simulink model "ddc_bpm_476_066_bak6"  (Simulink 7.8)
settings: Solver=ode45  StartTime=0.0  StopTime=2.56e-3  RelTol=1e-3
undefined symbols (not defined in the file): dt_sim, frev_476, Fs_adc, xlipgetpartsetting
libraries: xbsIndex_r4 x615, simulink x3
(part 6 of 6)

== system ddc_bpm_476_066_bak6/delta-sigma_tbt/unsigned2signed1 ==
  s_data : Inport
  u_data : Inport  Port=2
  Concat : xbsIndex_r4/Concat  num_inputs=2  dbl_ovrd=off  block_type=concat
  Convert : xbsIndex_r4/Convert  gui_display_data_type=Fixed-point  arith_type="Signed  (2's comp)"  n_bits=24  bin_pt=23  float_type=Single  exp_bits=8  fraction_bits=24  quantization=Truncate  overflow=Flag as error  en=off  latency=0  dbl_ovrd=off  pipeline=off  block_type=convert
  Reinterpret : xbsIndex_r4/Reinterpret  force_arith_type=on  arith_type="Signed  (2's comp)"  force_bin_pt=on  bin_pt=23  block_type=reinterpret
  Reinterpret1 : xbsIndex_r4/Reinterpret  force_arith_type=on  arith_type=Unsigned  force_bin_pt=on  bin_pt=0  block_type=reinterpret
  Reinterpret2 : xbsIndex_r4/Reinterpret  force_arith_type=on  arith_type=Unsigned  force_bin_pt=on  bin_pt=0  block_type=reinterpret
  data_out : Outport
  wires:
  Concat/1 -> Reinterpret/1
  Reinterpret2/1 -> Concat/1
  s_data/1 -> Reinterpret2/1
  Reinterpret/1 -> Convert/1
  u_data/1 -> Reinterpret1/1
  Reinterpret1/1 -> Concat/2
  Convert/1 -> data_out/1

== system ddc_bpm_476_066_bak6/delta-sigma_tbt/unsigned2signed2 ==
  s_data : Inport
  u_data : Inport  Port=2
  Concat : xbsIndex_r4/Concat  num_inputs=2  dbl_ovrd=off  block_type=concat
  Convert : xbsIndex_r4/Convert  gui_display_data_type=Fixed-point  arith_type="Signed  (2's comp)"  n_bits=24  bin_pt=23  float_type=Single  exp_bits=8  fraction_bits=24  quantization=Truncate  overflow=Flag as error  en=off  latency=0  dbl_ovrd=off  pipeline=off  block_type=convert
  Reinterpret : xbsIndex_r4/Reinterpret  force_arith_type=on  arith_type="Signed  (2's comp)"  force_bin_pt=on  bin_pt=23  block_type=reinterpret
  Reinterpret1 : xbsIndex_r4/Reinterpret  force_arith_type=on  arith_type=Unsigned  force_bin_pt=on  bin_pt=0  block_type=reinterpret
  Reinterpret2 : xbsIndex_r4/Reinterpret  force_arith_type=on  arith_type=Unsigned  force_bin_pt=on  bin_pt=0  block_type=reinterpret
  data_out : Outport
  wires:
  Concat/1 -> Reinterpret/1
  Reinterpret2/1 -> Concat/1
  s_data/1 -> Reinterpret2/1
  Reinterpret/1 -> Convert/1
  u_data/1 -> Reinterpret1/1
  Reinterpret1/1 -> Concat/2
  Convert/1 -> data_out/1

== system ddc_bpm_476_066_bak6/delta-sigma_tbt/unsigned2signed3 ==
  s_data : Inport
  u_data : Inport  Port=2
  Concat : xbsIndex_r4/Concat  num_inputs=2  dbl_ovrd=off  block_type=concat
  Convert : xbsIndex_r4/Convert  gui_display_data_type=Fixed-point  arith_type="Signed  (2's comp)"  n_bits=24  bin_pt=23  float_type=Single  exp_bits=8  fraction_bits=24  quantization=Truncate  overflow=Flag as error  en=off  latency=0  dbl_ovrd=off  pipeline=off  block_type=convert
  Reinterpret : xbsIndex_r4/Reinterpret  force_arith_type=on  arith_type="Signed  (2's comp)"  force_bin_pt=on  bin_pt=23  block_type=reinterpret
  Reinterpret1 : xbsIndex_r4/Reinterpret  force_arith_type=on  arith_type=Unsigned  force_bin_pt=on  bin_pt=0  block_type=reinterpret
  Reinterpret2 : xbsIndex_r4/Reinterpret  force_arith_type=on  arith_type=Unsigned  force_bin_pt=on  bin_pt=0  block_type=reinterpret
  data_out : Outport
  wires:
  Concat/1 -> Reinterpret/1
  Reinterpret2/1 -> Concat/1
  s_data/1 -> Reinterpret2/1
  Reinterpret/1 -> Convert/1
  u_data/1 -> Reinterpret1/1
  Reinterpret1/1 -> Concat/2
  Convert/1 -> data_out/1

== system ddc_bpm_476_066_bak6/Channel0_tbt/DDC/Mixer ==
  din_q : Inport
  din_i : Inport  Port=2
  en : Inport  Port=3
  dds_valid : Inport  Port=4
  dds_cosine : Inport  Port=5
  dds_msine : Inport  Port=6
  ComplexMult : xbsIndex_r4/Complex Multiplier 5.0   hasatlast=off  hasatuser=off  atuserwidth=1  hasbtlast=off  hasbtuser=off  btuserwidth=1  multtype=Use_Mults  optimizegoal=Performance  flowcontrol=NonBlocking  outputwidth=24  roundmode=Truncate  hasctrltlast=off  hasctrltuser=off  ctrltuserwidth=1  outtlastbehv=Null  latencyconfig=Manual  minimumlatency=6  aclken=off  aresetn=off  trim_axipin_name=on  aportwidth=63  bportwidth=63  ip_name=Complex Multiplier  ip_version=5.0  dsptool_ready=true  ipcore_usecache=true  ipcore_useipmodelcache=true  ipcore_verbose=false  ipcore_latency_parameter='minimumlatency'  wrapper_available=true  port_translation_map={ 'aclken' => 'en', 'aresetn' => 'rst'}  structural_sim=false  block_type=cmpy_v5_0
  Convert1 : xbsIndex_r4/Convert  gui_display_data_type=Fixed-point  arith_type="Signed  (2's comp)"  n_bits=24  bin_pt=22  float_type=Single  exp_bits=8  fraction_bits=24  quantization=Truncate  overflow=Flag as error  en=off  latency=0  dbl_ovrd=off  pipeline=off  block_type=convert
  Convert2 : xbsIndex_r4/Convert  gui_display_data_type=Fixed-point  arith_type="Signed  (2's comp)"  n_bits=24  bin_pt=22  float_type=Single  exp_bits=8  fraction_bits=24  quantization=Truncate  overflow=Flag as error  en=off  latency=0  dbl_ovrd=off  pipeline=off  block_type=convert
  DataReg_En : Subsystem
  DataReg_En1 : Subsystem
  Delay : xbsIndex_r4/Delay  rst=off  infoeditControl=Selection of Reset will increase slice count due to use of real FFs and instead of SRLs  en=off  latency=0  dbl_ovrd=off  reg_retiming=off  block_type=delay
      settings: infoedit=Hardware notes: A delay line is a chain, each link of which is an SRL16 followed by a flip-flop. If register retiming is enabled, the delay line is a chain of flip-flops.  xl_area=[7 14 0 0 0 0 0]  block_version=VER_STRING_GOES_HERE
  Delay1 : xbsIndex_r4/Delay  rst=off  infoeditControl=Selection of Reset will increase slice count due to use of real FFs and instead of SRLs  en=off  latency=0  dbl_ovrd=off  reg_retiming=off  block_type=delay
      settings: infoedit=Hardware notes: A delay line is a chain, each link of which is an SRL16 followed by a flip-flop. If register retiming is enabled, the delay line is a chain of flip-flops.  xl_area=[7 14 0 0 0 0 0]  block_version=VER_STRING_GOES_HERE
  Delay{2..3,6..7} (4 alike) : xbsIndex_r4/Delay  rst=off  infoeditControl=Selection of Reset will increase slice count due to use of real FFs and instead of SRLs  en=on  latency=1  dbl_ovrd=off  reg_retiming=off  block_type=delay
  Reinterpret : xbsIndex_r4/Reinterpret  force_arith_type=off  arith_type=Unsigned  force_bin_pt=off  bin_pt=22  block_type=reinterpret
  Reinterpret1 : xbsIndex_r4/Reinterpret  force_arith_type=off  arith_type=Unsigned  force_bin_pt=off  bin_pt=22  block_type=reinterpret
  Q : Outport
  I : Outport  Port=2
  valid_out : Outport  Port=3
  wires:
  din_q/1 -> DataReg_En/1(Din)
  DataReg_En/1(Dout) -> Delay/1
  din_i/1 -> DataReg_En1/1(Din)
  DataReg_En1/1(Dout) -> Delay1/1
  en/1 -> DataReg_En/2(en), DataReg_En1/2(en)
  dds_cosine/1 -> Delay3/1
  dds_msine/1 -> Delay2/1
  Delay3/1 -> ComplexMult/3  "a_r"
  Delay6/1 -> Q/1
  Delay2/1 -> ComplexMult/2  "a_i"
  ComplexMult/2 -> Reinterpret/1
  ComplexMult/3 -> Reinterpret1/1
  ComplexMult/1 -> Delay7/2, Delay6/2
  Delay1/1 -> ComplexMult/6  "b_r"
  Delay/1 -> ComplexMult/5  "b_i"
  DataReg_En/2(Valid) -> ComplexMult/4
  Delay7/1 -> I/1
  DataReg_En1/2(Valid) -> valid_out/1
  Convert1/1 -> Delay7/1
  Convert2/1 -> Delay6/1
  Reinterpret/1 -> Convert2/1
  Reinterpret1/1 -> Convert1/1
  dds_valid/1 -> Delay2/2, Delay3/2, ComplexMult/1

== system ddc_bpm_476_066_bak6/Channel0_tbt/decim35/Cast1 ==
  data_in : Inport
  en : Inport  Port=2
  Register : xbsIndex_r4/Register  init=0  rst=off  en=on  dbl_ovrd=off  block_type=register
      settings: xl_area=[0, 0, 0, 0, 0, 0, 0]  block_version=VER_STRING_GOES_HERE
  Register1 : xbsIndex_r4/Register  init=0  rst=off  en=off  dbl_ovrd=off  block_type=register
      settings: xl_area=[0, 0, 0, 0, 0, 0, 0]  block_version=VER_STRING_GOES_HERE
  format1 : Subsystem
  out : Outport
  valid : Outport  Port=2
  wires:
  format1/1(dout) -> Register/1
  Register/1 -> out/1
  data_in/1 -> format1/1(din)
  en/1 -> Register/2, Register1/1
  Register1/1 -> valid/1

== system ddc_bpm_476_066_bak6/Channel0_tbt/decim35/Cast4 ==
  data_in : Inport
  en : Inport  Port=2
  Register : xbsIndex_r4/Register  init=0  rst=off  en=on  dbl_ovrd=off  block_type=register
      settings: xl_area=[0, 0, 0, 0, 0, 0, 0]  block_version=VER_STRING_GOES_HERE
  Register1 : xbsIndex_r4/Register  init=0  rst=off  en=off  dbl_ovrd=off  block_type=register
      settings: xl_area=[0, 0, 0, 0, 0, 0, 0]  block_version=VER_STRING_GOES_HERE
  format1 : Subsystem
  out : Outport
  valid : Outport  Port=2
  wires:
  format1/1(dout) -> Register/1
  Register/1 -> out/1
  data_in/1 -> format1/1(din)
  en/1 -> Register/2, Register1/1
  Register1/1 -> valid/1

== system ddc_bpm_476_066_bak6/Channel1_tbt/DDC/Mixer ==
  din_q : Inport
  din_i : Inport  Port=2
  en : Inport  Port=3
  dds_valid : Inport  Port=4
  dds_cosine : Inport  Port=5
  dds_msine : Inport  Port=6
  ComplexMult : xbsIndex_r4/Complex Multiplier 5.0   hasatlast=off  hasatuser=off  atuserwidth=1  hasbtlast=off  hasbtuser=off  btuserwidth=1  multtype=Use_Mults  optimizegoal=Performance  flowcontrol=NonBlocking  outputwidth=24  roundmode=Truncate  hasctrltlast=off  hasctrltuser=off  ctrltuserwidth=1  outtlastbehv=Null  latencyconfig=Manual  minimumlatency=6  aclken=off  aresetn=off  trim_axipin_name=on  aportwidth=63  bportwidth=63  ip_name=Complex Multiplier  ip_version=5.0  dsptool_ready=true  ipcore_usecache=true  ipcore_useipmodelcache=true  ipcore_verbose=false  ipcore_latency_parameter='minimumlatency'  wrapper_available=true  port_translation_map={ 'aclken' => 'en', 'aresetn' => 'rst'}  structural_sim=false  block_type=cmpy_v5_0
  Convert1 : xbsIndex_r4/Convert  gui_display_data_type=Fixed-point  arith_type="Signed  (2's comp)"  n_bits=24  bin_pt=22  float_type=Single  exp_bits=8  fraction_bits=24  quantization=Truncate  overflow=Flag as error  en=off  latency=0  dbl_ovrd=off  pipeline=off  block_type=convert
  Convert2 : xbsIndex_r4/Convert  gui_display_data_type=Fixed-point  arith_type="Signed  (2's comp)"  n_bits=24  bin_pt=22  float_type=Single  exp_bits=8  fraction_bits=24  quantization=Truncate  overflow=Flag as error  en=off  latency=0  dbl_ovrd=off  pipeline=off  block_type=convert
  DataReg_En : Subsystem
  DataReg_En1 : Subsystem
  Delay : xbsIndex_r4/Delay  rst=off  infoeditControl=Selection of Reset will increase slice count due to use of real FFs and instead of SRLs  en=off  latency=0  dbl_ovrd=off  reg_retiming=off  block_type=delay
      settings: infoedit=Hardware notes: A delay line is a chain, each link of which is an SRL16 followed by a flip-flop. If register retiming is enabled, the delay line is a chain of flip-flops.  xl_area=[7 14 0 0 0 0 0]  block_version=VER_STRING_GOES_HERE
  Delay1 : xbsIndex_r4/Delay  rst=off  infoeditControl=Selection of Reset will increase slice count due to use of real FFs and instead of SRLs  en=off  latency=0  dbl_ovrd=off  reg_retiming=off  block_type=delay
      settings: infoedit=Hardware notes: A delay line is a chain, each link of which is an SRL16 followed by a flip-flop. If register retiming is enabled, the delay line is a chain of flip-flops.  xl_area=[7 14 0 0 0 0 0]  block_version=VER_STRING_GOES_HERE
  Delay{2..3,6..7} (4 alike) : xbsIndex_r4/Delay  rst=off  infoeditControl=Selection of Reset will increase slice count due to use of real FFs and instead of SRLs  en=on  latency=1  dbl_ovrd=off  reg_retiming=off  block_type=delay
  Reinterpret : xbsIndex_r4/Reinterpret  force_arith_type=off  arith_type=Unsigned  force_bin_pt=off  bin_pt=22  block_type=reinterpret
  Reinterpret1 : xbsIndex_r4/Reinterpret  force_arith_type=off  arith_type=Unsigned  force_bin_pt=off  bin_pt=22  block_type=reinterpret
  Q : Outport
  I : Outport  Port=2
  valid_out : Outport  Port=3
  wires:
  din_q/1 -> DataReg_En/1(Din)
  DataReg_En/1(Dout) -> Delay/1
  din_i/1 -> DataReg_En1/1(Din)
  DataReg_En1/1(Dout) -> Delay1/1
  en/1 -> DataReg_En/2(en), DataReg_En1/2(en)
  dds_cosine/1 -> Delay3/1
  dds_msine/1 -> Delay2/1
  Delay3/1 -> ComplexMult/3  "a_r"
  Delay6/1 -> Q/1
  Delay2/1 -> ComplexMult/2  "a_i"
  ComplexMult/2 -> Reinterpret/1
  ComplexMult/3 -> Reinterpret1/1
  ComplexMult/1 -> Delay7/2, Delay6/2
  Delay1/1 -> ComplexMult/6  "b_r"
  Delay/1 -> ComplexMult/5  "b_i"
  DataReg_En/2(Valid) -> ComplexMult/4
  Delay7/1 -> I/1
  DataReg_En1/2(Valid) -> valid_out/1
  Convert1/1 -> Delay7/1
  Convert2/1 -> Delay6/1
  Reinterpret/1 -> Convert2/1
  Reinterpret1/1 -> Convert1/1
  dds_valid/1 -> Delay2/2, Delay3/2, ComplexMult/1

== system ddc_bpm_476_066_bak6/Channel1_tbt/decim35/Cast1 ==
  data_in : Inport
  en : Inport  Port=2
  Register : xbsIndex_r4/Register  init=0  rst=off  en=on  dbl_ovrd=off  block_type=register
      settings: xl_area=[0, 0, 0, 0, 0, 0, 0]  block_version=VER_STRING_GOES_HERE
  Register1 : xbsIndex_r4/Register  init=0  rst=off  en=off  dbl_ovrd=off  block_type=register
      settings: xl_area=[0, 0, 0, 0, 0, 0, 0]  block_version=VER_STRING_GOES_HERE
  format1 : Subsystem
  out : Outport
  valid : Outport  Port=2
  wires:
  format1/1(dout) -> Register/1
  Register/1 -> out/1
  data_in/1 -> format1/1(din)
  en/1 -> Register/2, Register1/1
  Register1/1 -> valid/1

== system ddc_bpm_476_066_bak6/Channel1_tbt/decim35/Cast4 ==
  data_in : Inport
  en : Inport  Port=2
  Register : xbsIndex_r4/Register  init=0  rst=off  en=on  dbl_ovrd=off  block_type=register
      settings: xl_area=[0, 0, 0, 0, 0, 0, 0]  block_version=VER_STRING_GOES_HERE
  Register1 : xbsIndex_r4/Register  init=0  rst=off  en=off  dbl_ovrd=off  block_type=register
      settings: xl_area=[0, 0, 0, 0, 0, 0, 0]  block_version=VER_STRING_GOES_HERE
  format1 : Subsystem
  out : Outport
  valid : Outport  Port=2
  wires:
  format1/1(dout) -> Register/1
  Register/1 -> out/1
  data_in/1 -> format1/1(din)
  en/1 -> Register/2, Register1/1
  Register1/1 -> valid/1

== system ddc_bpm_476_066_bak6/Channel2_tbt/DDC/Mixer ==
  din_q : Inport
  din_i : Inport  Port=2
  en : Inport  Port=3
  dds_valid : Inport  Port=4
  dds_cosine : Inport  Port=5
  dds_msine : Inport  Port=6
  ComplexMult : xbsIndex_r4/Complex Multiplier 5.0   hasatlast=off  hasatuser=off  atuserwidth=1  hasbtlast=off  hasbtuser=off  btuserwidth=1  multtype=Use_Mults  optimizegoal=Performance  flowcontrol=NonBlocking  outputwidth=24  roundmode=Truncate  hasctrltlast=off  hasctrltuser=off  ctrltuserwidth=1  outtlastbehv=Null  latencyconfig=Manual  minimumlatency=6  aclken=off  aresetn=off  trim_axipin_name=on  aportwidth=63  bportwidth=63  ip_name=Complex Multiplier  ip_version=5.0  dsptool_ready=true  ipcore_usecache=true  ipcore_useipmodelcache=true  ipcore_verbose=false  ipcore_latency_parameter='minimumlatency'  wrapper_available=true  port_translation_map={ 'aclken' => 'en', 'aresetn' => 'rst'}  structural_sim=false  block_type=cmpy_v5_0
  Convert1 : xbsIndex_r4/Convert  gui_display_data_type=Fixed-point  arith_type="Signed  (2's comp)"  n_bits=24  bin_pt=22  float_type=Single  exp_bits=8  fraction_bits=24  quantization=Truncate  overflow=Flag as error  en=off  latency=0  dbl_ovrd=off  pipeline=off  block_type=convert
  Convert2 : xbsIndex_r4/Convert  gui_display_data_type=Fixed-point  arith_type="Signed  (2's comp)"  n_bits=24  bin_pt=22  float_type=Single  exp_bits=8  fraction_bits=24  quantization=Truncate  overflow=Flag as error  en=off  latency=0  dbl_ovrd=off  pipeline=off  block_type=convert
  DataReg_En : Subsystem
  DataReg_En1 : Subsystem
  Delay : xbsIndex_r4/Delay  rst=off  infoeditControl=Selection of Reset will increase slice count due to use of real FFs and instead of SRLs  en=off  latency=0  dbl_ovrd=off  reg_retiming=off  block_type=delay
      settings: infoedit=Hardware notes: A delay line is a chain, each link of which is an SRL16 followed by a flip-flop. If register retiming is enabled, the delay line is a chain of flip-flops.  xl_area=[7 14 0 0 0 0 0]  block_version=VER_STRING_GOES_HERE
  Delay1 : xbsIndex_r4/Delay  rst=off  infoeditControl=Selection of Reset will increase slice count due to use of real FFs and instead of SRLs  en=off  latency=0  dbl_ovrd=off  reg_retiming=off  block_type=delay
      settings: infoedit=Hardware notes: A delay line is a chain, each link of which is an SRL16 followed by a flip-flop. If register retiming is enabled, the delay line is a chain of flip-flops.  xl_area=[7 14 0 0 0 0 0]  block_version=VER_STRING_GOES_HERE
  Delay{2..3,6..7} (4 alike) : xbsIndex_r4/Delay  rst=off  infoeditControl=Selection of Reset will increase slice count due to use of real FFs and instead of SRLs  en=on  latency=1  dbl_ovrd=off  reg_retiming=off  block_type=delay
  Reinterpret : xbsIndex_r4/Reinterpret  force_arith_type=off  arith_type=Unsigned  force_bin_pt=off  bin_pt=22  block_type=reinterpret
  Reinterpret1 : xbsIndex_r4/Reinterpret  force_arith_type=off  arith_type=Unsigned  force_bin_pt=off  bin_pt=22  block_type=reinterpret
  Q : Outport
  I : Outport  Port=2
  valid_out : Outport  Port=3
  wires:
  din_q/1 -> DataReg_En/1(Din)
  DataReg_En/1(Dout) -> Delay/1
  din_i/1 -> DataReg_En1/1(Din)
  DataReg_En1/1(Dout) -> Delay1/1
  en/1 -> DataReg_En/2(en), DataReg_En1/2(en)
  dds_cosine/1 -> Delay3/1
  dds_msine/1 -> Delay2/1
  Delay3/1 -> ComplexMult/3  "a_r"
  Delay6/1 -> Q/1
  Delay2/1 -> ComplexMult/2  "a_i"
  ComplexMult/2 -> Reinterpret/1
  ComplexMult/3 -> Reinterpret1/1
  ComplexMult/1 -> Delay7/2, Delay6/2
  Delay1/1 -> ComplexMult/6  "b_r"
  Delay/1 -> ComplexMult/5  "b_i"
  DataReg_En/2(Valid) -> ComplexMult/4
  Delay7/1 -> I/1
  DataReg_En1/2(Valid) -> valid_out/1
  Convert1/1 -> Delay7/1
  Convert2/1 -> Delay6/1
  Reinterpret/1 -> Convert2/1
  Reinterpret1/1 -> Convert1/1
  dds_valid/1 -> Delay2/2, Delay3/2, ComplexMult/1

== system ddc_bpm_476_066_bak6/Channel2_tbt/decim35/Cast1 ==
  data_in : Inport
  en : Inport  Port=2
  Register : xbsIndex_r4/Register  init=0  rst=off  en=on  dbl_ovrd=off  block_type=register
      settings: xl_area=[0, 0, 0, 0, 0, 0, 0]  block_version=VER_STRING_GOES_HERE
  Register1 : xbsIndex_r4/Register  init=0  rst=off  en=off  dbl_ovrd=off  block_type=register
      settings: xl_area=[0, 0, 0, 0, 0, 0, 0]  block_version=VER_STRING_GOES_HERE
  format1 : Subsystem
  out : Outport
  valid : Outport  Port=2
  wires:
  format1/1(dout) -> Register/1
  Register/1 -> out/1
  data_in/1 -> format1/1(din)
  en/1 -> Register/2, Register1/1
  Register1/1 -> valid/1

== system ddc_bpm_476_066_bak6/Channel2_tbt/decim35/Cast4 ==
  data_in : Inport
  en : Inport  Port=2
  Register : xbsIndex_r4/Register  init=0  rst=off  en=on  dbl_ovrd=off  block_type=register
      settings: xl_area=[0, 0, 0, 0, 0, 0, 0]  block_version=VER_STRING_GOES_HERE
  Register1 : xbsIndex_r4/Register  init=0  rst=off  en=off  dbl_ovrd=off  block_type=register
      settings: xl_area=[0, 0, 0, 0, 0, 0, 0]  block_version=VER_STRING_GOES_HERE
  format1 : Subsystem
  out : Outport
  valid : Outport  Port=2
  wires:
  format1/1(dout) -> Register/1
  Register/1 -> out/1
  data_in/1 -> format1/1(din)
  en/1 -> Register/2, Register1/1
  Register1/1 -> valid/1

== system ddc_bpm_476_066_bak6/Channel3_tbt/DDC/Mixer ==
  din_q : Inport
  din_i : Inport  Port=2
  en : Inport  Port=3
  dds_valid : Inport  Port=4
  dds_cosine : Inport  Port=5
  dds_msine : Inport  Port=6
  ComplexMult : xbsIndex_r4/Complex Multiplier 5.0   hasatlast=off  hasatuser=off  atuserwidth=1  hasbtlast=off  hasbtuser=off  btuserwidth=1  multtype=Use_Mults  optimizegoal=Performance  flowcontrol=NonBlocking  outputwidth=24  roundmode=Truncate  hasctrltlast=off  hasctrltuser=off  ctrltuserwidth=1  outtlastbehv=Null  latencyconfig=Manual  minimumlatency=6  aclken=off  aresetn=off  trim_axipin_name=on  aportwidth=63  bportwidth=63  ip_name=Complex Multiplier  ip_version=5.0  dsptool_ready=true  ipcore_usecache=true  ipcore_useipmodelcache=true  ipcore_verbose=false  ipcore_latency_parameter='minimumlatency'  wrapper_available=true  port_translation_map={ 'aclken' => 'en', 'aresetn' => 'rst'}  structural_sim=false  block_type=cmpy_v5_0
  Convert1 : xbsIndex_r4/Convert  gui_display_data_type=Fixed-point  arith_type="Signed  (2's comp)"  n_bits=24  bin_pt=22  float_type=Single  exp_bits=8  fraction_bits=24  quantization=Truncate  overflow=Flag as error  en=off  latency=0  dbl_ovrd=off  pipeline=off  block_type=convert
  Convert2 : xbsIndex_r4/Convert  gui_display_data_type=Fixed-point  arith_type="Signed  (2's comp)"  n_bits=24  bin_pt=22  float_type=Single  exp_bits=8  fraction_bits=24  quantization=Truncate  overflow=Flag as error  en=off  latency=0  dbl_ovrd=off  pipeline=off  block_type=convert
  DataReg_En : Subsystem
  DataReg_En1 : Subsystem
  Delay : xbsIndex_r4/Delay  rst=off  infoeditControl=Selection of Reset will increase slice count due to use of real FFs and instead of SRLs  en=off  latency=0  dbl_ovrd=off  reg_retiming=off  block_type=delay
      settings: infoedit=Hardware notes: A delay line is a chain, each link of which is an SRL16 followed by a flip-flop. If register retiming is enabled, the delay line is a chain of flip-flops.  xl_area=[7 14 0 0 0 0 0]  block_version=VER_STRING_GOES_HERE
  Delay1 : xbsIndex_r4/Delay  rst=off  infoeditControl=Selection of Reset will increase slice count due to use of real FFs and instead of SRLs  en=off  latency=0  dbl_ovrd=off  reg_retiming=off  block_type=delay
      settings: infoedit=Hardware notes: A delay line is a chain, each link of which is an SRL16 followed by a flip-flop. If register retiming is enabled, the delay line is a chain of flip-flops.  xl_area=[7 14 0 0 0 0 0]  block_version=VER_STRING_GOES_HERE
  Delay{2..3,6..7} (4 alike) : xbsIndex_r4/Delay  rst=off  infoeditControl=Selection of Reset will increase slice count due to use of real FFs and instead of SRLs  en=on  latency=1  dbl_ovrd=off  reg_retiming=off  block_type=delay
  Reinterpret : xbsIndex_r4/Reinterpret  force_arith_type=off  arith_type=Unsigned  force_bin_pt=off  bin_pt=22  block_type=reinterpret
  Reinterpret1 : xbsIndex_r4/Reinterpret  force_arith_type=off  arith_type=Unsigned  force_bin_pt=off  bin_pt=22  block_type=reinterpret
  Q : Outport
  I : Outport  Port=2
  valid_out : Outport  Port=3
  wires:
  din_q/1 -> DataReg_En/1(Din)
  DataReg_En/1(Dout) -> Delay/1
  din_i/1 -> DataReg_En1/1(Din)
  DataReg_En1/1(Dout) -> Delay1/1
  en/1 -> DataReg_En/2(en), DataReg_En1/2(en)
  dds_cosine/1 -> Delay3/1
  dds_msine/1 -> Delay2/1
  Delay3/1 -> ComplexMult/3  "a_r"
  Delay6/1 -> Q/1
  Delay2/1 -> ComplexMult/2  "a_i"
  ComplexMult/2 -> Reinterpret/1
  ComplexMult/3 -> Reinterpret1/1
  ComplexMult/1 -> Delay7/2, Delay6/2
  Delay1/1 -> ComplexMult/6  "b_r"
  Delay/1 -> ComplexMult/5  "b_i"
  DataReg_En/2(Valid) -> ComplexMult/4
  Delay7/1 -> I/1
  DataReg_En1/2(Valid) -> valid_out/1
  Convert1/1 -> Delay7/1
  Convert2/1 -> Delay6/1
  Reinterpret/1 -> Convert2/1
  Reinterpret1/1 -> Convert1/1
  dds_valid/1 -> Delay2/2, Delay3/2, ComplexMult/1

== system ddc_bpm_476_066_bak6/Channel3_tbt/decim35/Cast1 ==
  data_in : Inport
  en : Inport  Port=2
  Register : xbsIndex_r4/Register  init=0  rst=off  en=on  dbl_ovrd=off  block_type=register
      settings: xl_area=[0, 0, 0, 0, 0, 0, 0]  block_version=VER_STRING_GOES_HERE
  Register1 : xbsIndex_r4/Register  init=0  rst=off  en=off  dbl_ovrd=off  block_type=register
      settings: xl_area=[0, 0, 0, 0, 0, 0, 0]  block_version=VER_STRING_GOES_HERE
  format1 : Subsystem
  out : Outport
  valid : Outport  Port=2
  wires:
  format1/1(dout) -> Register/1
  Register/1 -> out/1
  data_in/1 -> format1/1(din)
  en/1 -> Register/2, Register1/1
  Register1/1 -> valid/1

== system ddc_bpm_476_066_bak6/Channel3_tbt/decim35/Cast4 ==
  data_in : Inport
  en : Inport  Port=2
  Register : xbsIndex_r4/Register  init=0  rst=off  en=on  dbl_ovrd=off  block_type=register
      settings: xl_area=[0, 0, 0, 0, 0, 0, 0]  block_version=VER_STRING_GOES_HERE
  Register1 : xbsIndex_r4/Register  init=0  rst=off  en=off  dbl_ovrd=off  block_type=register
      settings: xl_area=[0, 0, 0, 0, 0, 0, 0]  block_version=VER_STRING_GOES_HERE
  format1 : Subsystem
  out : Outport
  valid : Outport  Port=2
  wires:
  format1/1(dout) -> Register/1
  Register/1 -> out/1
  data_in/1 -> format1/1(din)
  en/1 -> Register/2, Register1/1
  Register1/1 -> valid/1

== system ddc_bpm_476_066_bak6/Decim_monit/Cast/format1 ==
  din : Inport
  Convert : xbsIndex_r4/Convert  gui_display_data_type=Fixed-point  arith_type="Signed  (2's comp)"  n_bits=24  bin_pt=22  float_type=Single  exp_bits=8  fraction_bits=24  quantization="Round  (unbiased: +/- Inf)"  overflow=Flag as error  en=off  latency=0  dbl_ovrd=off  pipeline=off  block_type=convert
  Reinterpret : xbsIndex_r4/Reinterpret  force_arith_type=on  arith_type="Signed  (2's comp)"  force_bin_pt=off  bin_pt=22  block_type=reinterpret
      settings: block_version=10.1
  dout : Outport
  wires:
  din/1 -> Reinterpret/1
  Convert/1 -> dout/1
  Reinterpret/1 -> Convert/1

== system ddc_bpm_476_066_bak6/Decim_monit/Cast1/format1 ==
  din : Inport
  Convert : xbsIndex_r4/Convert  gui_display_data_type=Fixed-point  arith_type="Signed  (2's comp)"  n_bits=24  bin_pt=22  float_type=Single  exp_bits=8  fraction_bits=24  quantization="Round  (unbiased: +/- Inf)"  overflow=Flag as error  en=off  latency=0  dbl_ovrd=off  pipeline=off  block_type=convert
  Reinterpret : xbsIndex_r4/Reinterpret  force_arith_type=on  arith_type="Signed  (2's comp)"  force_bin_pt=off  bin_pt=22  block_type=reinterpret
      settings: block_version=10.1
  dout : Outport
  wires:
  din/1 -> Reinterpret/1
  Convert/1 -> dout/1
  Reinterpret/1 -> Convert/1

== system ddc_bpm_476_066_bak6/Decim_monit/Cast2/format1 ==
  din : Inport
  Convert : xbsIndex_r4/Convert  gui_display_data_type=Fixed-point  arith_type="Signed  (2's comp)"  n_bits=24  bin_pt=22  float_type=Single  exp_bits=8  fraction_bits=24  quantization="Round  (unbiased: +/- Inf)"  overflow=Flag as error  en=off  latency=0  dbl_ovrd=off  pipeline=off  block_type=convert
  Reinterpret : xbsIndex_r4/Reinterpret  force_arith_type=on  arith_type="Signed  (2's comp)"  force_bin_pt=off  bin_pt=22  block_type=reinterpret
      settings: block_version=10.1
  dout : Outport
  wires:
  din/1 -> Reinterpret/1
  Convert/1 -> dout/1
  Reinterpret/1 -> Convert/1

== system ddc_bpm_476_066_bak6/Decim_monit/Cast3/format1 ==
  din : Inport
  Convert : xbsIndex_r4/Convert  gui_display_data_type=Fixed-point  arith_type="Signed  (2's comp)"  n_bits=24  bin_pt=22  float_type=Single  exp_bits=8  fraction_bits=24  quantization="Round  (unbiased: +/- Inf)"  overflow=Flag as error  en=off  latency=0  dbl_ovrd=off  pipeline=off  block_type=convert
  Reinterpret : xbsIndex_r4/Reinterpret  force_arith_type=on  arith_type="Signed  (2's comp)"  force_bin_pt=off  bin_pt=22  block_type=reinterpret
      settings: block_version=10.1
  dout : Outport
  wires:
  din/1 -> Reinterpret/1
  Convert/1 -> dout/1
  Reinterpret/1 -> Convert/1

== system ddc_bpm_476_066_bak6/Decim_monit/Cast4/format1 ==
  din : Inport
  Convert : xbsIndex_r4/Convert  gui_display_data_type=Fixed-point  arith_type="Signed  (2's comp)"  n_bits=24  bin_pt=22  float_type=Single  exp_bits=8  fraction_bits=24  quantization="Round  (unbiased: +/- Inf)"  overflow=Flag as error  en=off  latency=0  dbl_ovrd=off  pipeline=off  block_type=convert
  Reinterpret : xbsIndex_r4/Reinterpret  force_arith_type=on  arith_type="Signed  (2's comp)"  force_bin_pt=off  bin_pt=22  block_type=reinterpret
      settings: block_version=10.1
  dout : Outport
  wires:
  din/1 -> Reinterpret/1
  Convert/1 -> dout/1
  Reinterpret/1 -> Convert/1

== system ddc_bpm_476_066_bak6/Decim_monit/Cast5/format1 ==
  din : Inport
  Convert : xbsIndex_r4/Convert  gui_display_data_type=Fixed-point  arith_type="Signed  (2's comp)"  n_bits=24  bin_pt=22  float_type=Single  exp_bits=8  fraction_bits=24  quantization="Round  (unbiased: +/- Inf)"  overflow=Flag as error  en=off  latency=0  dbl_ovrd=off  pipeline=off  block_type=convert
  Reinterpret : xbsIndex_r4/Reinterpret  force_arith_type=on  arith_type="Signed  (2's comp)"  force_bin_pt=off  bin_pt=22  block_type=reinterpret
      settings: block_version=10.1
  dout : Outport
  wires:
  din/1 -> Reinterpret/1
  Convert/1 -> dout/1
  Reinterpret/1 -> Convert/1

== system ddc_bpm_476_066_bak6/Decim_monit/Cast6/format1 ==
  din : Inport
  Convert : xbsIndex_r4/Convert  gui_display_data_type=Fixed-point  arith_type="Signed  (2's comp)"  n_bits=24  bin_pt=22  float_type=Single  exp_bits=8  fraction_bits=24  quantization="Round  (unbiased: +/- Inf)"  overflow=Flag as error  en=off  latency=0  dbl_ovrd=off  pipeline=off  block_type=convert
  Reinterpret : xbsIndex_r4/Reinterpret  force_arith_type=on  arith_type="Signed  (2's comp)"  force_bin_pt=off  bin_pt=22  block_type=reinterpret
      settings: block_version=10.1
  dout : Outport
  wires:
  din/1 -> Reinterpret/1
  Convert/1 -> dout/1
  Reinterpret/1 -> Convert/1

== system ddc_bpm_476_066_bak6/Decim_monit/Cast7/format1 ==
  din : Inport
  Convert : xbsIndex_r4/Convert  gui_display_data_type=Fixed-point  arith_type="Signed  (2's comp)"  n_bits=24  bin_pt=22  float_type=Single  exp_bits=8  fraction_bits=24  quantization="Round  (unbiased: +/- Inf)"  overflow=Flag as error  en=off  latency=0  dbl_ovrd=off  pipeline=off  block_type=convert
  Reinterpret : xbsIndex_r4/Reinterpret  force_arith_type=on  arith_type="Signed  (2's comp)"  force_bin_pt=off  bin_pt=22  block_type=reinterpret
      settings: block_version=10.1
  dout : Outport
  wires:
  din/1 -> Reinterpret/1
  Convert/1 -> dout/1
  Reinterpret/1 -> Convert/1

== system ddc_bpm_476_066_bak6/Channel0_tbt/DDC/Mixer/DataReg_En ==
  Din : Inport
  en : Inport  Port=2
  Register : xbsIndex_r4/Register  init=0  rst=off  en=on  dbl_ovrd=off  block_type=register
      settings: block_version=VER_STRING_GOES_HERE
  Register1 : xbsIndex_r4/Register  init=0  rst=off  en=off  dbl_ovrd=off  block_type=register
      settings: block_version=VER_STRING_GOES_HERE
  Dout : Outport
  Valid : Outport  Port=2
  wires:
  Din/1 -> Register/1
  Register/1 -> Dout/1
  Register1/1 -> Valid/1
  en/1 -> Register1/1, Register/2

== system ddc_bpm_476_066_bak6/Channel0_tbt/DDC/Mixer/DataReg_En1 ==
  Din : Inport
  en : Inport  Port=2
  Register : xbsIndex_r4/Register  init=0  rst=off  en=on  dbl_ovrd=off  block_type=register
      settings: block_version=VER_STRING_GOES_HERE
  Register1 : xbsIndex_r4/Register  init=0  rst=off  en=off  dbl_ovrd=off  block_type=register
      settings: block_version=VER_STRING_GOES_HERE
  Dout : Outport
  Valid : Outport  Port=2
  wires:
  en/1 -> Register1/1, Register/2
  Register1/1 -> Valid/1
  Register/1 -> Dout/1
  Din/1 -> Register/1

== system ddc_bpm_476_066_bak6/Channel0_tbt/decim35/Cast1/format1 ==
  din : Inport
  Convert : xbsIndex_r4/Convert  gui_display_data_type=Fixed-point  arith_type="Signed  (2's comp)"  n_bits=24  bin_pt=22  float_type=Single  exp_bits=8  fraction_bits=24  quantization="Round  (unbiased: +/- Inf)"  overflow=Flag as error  en=off  latency=0  dbl_ovrd=off  pipeline=off  block_type=convert
  Reinterpret : xbsIndex_r4/Reinterpret  force_arith_type=on  arith_type="Signed  (2's comp)"  force_bin_pt=off  bin_pt=22  block_type=reinterpret
      settings: block_version=10.1
  dout : Outport
  wires:
  din/1 -> Reinterpret/1
  Convert/1 -> dout/1
  Reinterpret/1 -> Convert/1

== system ddc_bpm_476_066_bak6/Channel0_tbt/decim35/Cast4/format1 ==
  din : Inport
  Convert : xbsIndex_r4/Convert  gui_display_data_type=Fixed-point  arith_type="Signed  (2's comp)"  n_bits=24  bin_pt=22  float_type=Single  exp_bits=8  fraction_bits=24  quantization="Round  (unbiased: +/- Inf)"  overflow=Flag as error  en=off  latency=0  dbl_ovrd=off  pipeline=off  block_type=convert
  Reinterpret : xbsIndex_r4/Reinterpret  force_arith_type=on  arith_type="Signed  (2's comp)"  force_bin_pt=off  bin_pt=22  block_type=reinterpret
      settings: block_version=10.1
  dout : Outport
  wires:
  din/1 -> Reinterpret/1
  Convert/1 -> dout/1
  Reinterpret/1 -> Convert/1

== system ddc_bpm_476_066_bak6/Channel1_tbt/DDC/Mixer/DataReg_En ==
  Din : Inport
  en : Inport  Port=2
  Register : xbsIndex_r4/Register  init=0  rst=off  en=on  dbl_ovrd=off  block_type=register
      settings: block_version=VER_STRING_GOES_HERE
  Register1 : xbsIndex_r4/Register  init=0  rst=off  en=off  dbl_ovrd=off  block_type=register
      settings: block_version=VER_STRING_GOES_HERE
  Dout : Outport
  Valid : Outport  Port=2
  wires:
  Din/1 -> Register/1
  Register/1 -> Dout/1
  Register1/1 -> Valid/1
  en/1 -> Register1/1, Register/2

== system ddc_bpm_476_066_bak6/Channel1_tbt/DDC/Mixer/DataReg_En1 ==
  Din : Inport
  en : Inport  Port=2
  Register : xbsIndex_r4/Register  init=0  rst=off  en=on  dbl_ovrd=off  block_type=register
      settings: block_version=VER_STRING_GOES_HERE
  Register1 : xbsIndex_r4/Register  init=0  rst=off  en=off  dbl_ovrd=off  block_type=register
      settings: block_version=VER_STRING_GOES_HERE
  Dout : Outport
  Valid : Outport  Port=2
  wires:
  en/1 -> Register1/1, Register/2
  Register1/1 -> Valid/1
  Register/1 -> Dout/1
  Din/1 -> Register/1

== system ddc_bpm_476_066_bak6/Channel1_tbt/decim35/Cast1/format1 ==
  din : Inport
  Convert : xbsIndex_r4/Convert  gui_display_data_type=Fixed-point  arith_type="Signed  (2's comp)"  n_bits=24  bin_pt=22  float_type=Single  exp_bits=8  fraction_bits=24  quantization="Round  (unbiased: +/- Inf)"  overflow=Flag as error  en=off  latency=0  dbl_ovrd=off  pipeline=off  block_type=convert
  Reinterpret : xbsIndex_r4/Reinterpret  force_arith_type=on  arith_type="Signed  (2's comp)"  force_bin_pt=off  bin_pt=22  block_type=reinterpret
      settings: block_version=10.1
  dout : Outport
  wires:
  din/1 -> Reinterpret/1
  Convert/1 -> dout/1
  Reinterpret/1 -> Convert/1

== system ddc_bpm_476_066_bak6/Channel1_tbt/decim35/Cast4/format1 ==
  din : Inport
  Convert : xbsIndex_r4/Convert  gui_display_data_type=Fixed-point  arith_type="Signed  (2's comp)"  n_bits=24  bin_pt=22  float_type=Single  exp_bits=8  fraction_bits=24  quantization="Round  (unbiased: +/- Inf)"  overflow=Flag as error  en=off  latency=0  dbl_ovrd=off  pipeline=off  block_type=convert
  Reinterpret : xbsIndex_r4/Reinterpret  force_arith_type=on  arith_type="Signed  (2's comp)"  force_bin_pt=off  bin_pt=22  block_type=reinterpret
      settings: block_version=10.1
  dout : Outport
  wires:
  din/1 -> Reinterpret/1
  Convert/1 -> dout/1
  Reinterpret/1 -> Convert/1

== system ddc_bpm_476_066_bak6/Channel2_tbt/DDC/Mixer/DataReg_En ==
  Din : Inport
  en : Inport  Port=2
  Register : xbsIndex_r4/Register  init=0  rst=off  en=on  dbl_ovrd=off  block_type=register
      settings: block_version=VER_STRING_GOES_HERE
  Register1 : xbsIndex_r4/Register  init=0  rst=off  en=off  dbl_ovrd=off  block_type=register
      settings: block_version=VER_STRING_GOES_HERE
  Dout : Outport
  Valid : Outport  Port=2
  wires:
  Din/1 -> Register/1
  Register/1 -> Dout/1
  Register1/1 -> Valid/1
  en/1 -> Register1/1, Register/2

== system ddc_bpm_476_066_bak6/Channel2_tbt/DDC/Mixer/DataReg_En1 ==
  Din : Inport
  en : Inport  Port=2
  Register : xbsIndex_r4/Register  init=0  rst=off  en=on  dbl_ovrd=off  block_type=register
      settings: block_version=VER_STRING_GOES_HERE
  Register1 : xbsIndex_r4/Register  init=0  rst=off  en=off  dbl_ovrd=off  block_type=register
      settings: block_version=VER_STRING_GOES_HERE
  Dout : Outport
  Valid : Outport  Port=2
  wires:
  en/1 -> Register1/1, Register/2
  Register1/1 -> Valid/1
  Register/1 -> Dout/1
  Din/1 -> Register/1

== system ddc_bpm_476_066_bak6/Channel2_tbt/decim35/Cast1/format1 ==
  din : Inport
  Convert : xbsIndex_r4/Convert  gui_display_data_type=Fixed-point  arith_type="Signed  (2's comp)"  n_bits=24  bin_pt=22  float_type=Single  exp_bits=8  fraction_bits=24  quantization="Round  (unbiased: +/- Inf)"  overflow=Flag as error  en=off  latency=0  dbl_ovrd=off  pipeline=off  block_type=convert
  Reinterpret : xbsIndex_r4/Reinterpret  force_arith_type=on  arith_type="Signed  (2's comp)"  force_bin_pt=off  bin_pt=22  block_type=reinterpret
      settings: block_version=10.1
  dout : Outport
  wires:
  din/1 -> Reinterpret/1
  Convert/1 -> dout/1
  Reinterpret/1 -> Convert/1

== system ddc_bpm_476_066_bak6/Channel2_tbt/decim35/Cast4/format1 ==
  din : Inport
  Convert : xbsIndex_r4/Convert  gui_display_data_type=Fixed-point  arith_type="Signed  (2's comp)"  n_bits=24  bin_pt=22  float_type=Single  exp_bits=8  fraction_bits=24  quantization="Round  (unbiased: +/- Inf)"  overflow=Flag as error  en=off  latency=0  dbl_ovrd=off  pipeline=off  block_type=convert
  Reinterpret : xbsIndex_r4/Reinterpret  force_arith_type=on  arith_type="Signed  (2's comp)"  force_bin_pt=off  bin_pt=22  block_type=reinterpret
      settings: block_version=10.1
  dout : Outport
  wires:
  din/1 -> Reinterpret/1
  Convert/1 -> dout/1
  Reinterpret/1 -> Convert/1

== system ddc_bpm_476_066_bak6/Channel3_tbt/DDC/Mixer/DataReg_En ==
  Din : Inport
  en : Inport  Port=2
  Register : xbsIndex_r4/Register  init=0  rst=off  en=on  dbl_ovrd=off  block_type=register
      settings: block_version=VER_STRING_GOES_HERE
  Register1 : xbsIndex_r4/Register  init=0  rst=off  en=off  dbl_ovrd=off  block_type=register
      settings: block_version=VER_STRING_GOES_HERE
  Dout : Outport
  Valid : Outport  Port=2
  wires:
  Din/1 -> Register/1
  Register/1 -> Dout/1
  Register1/1 -> Valid/1
  en/1 -> Register1/1, Register/2

== system ddc_bpm_476_066_bak6/Channel3_tbt/DDC/Mixer/DataReg_En1 ==
  Din : Inport
  en : Inport  Port=2
  Register : xbsIndex_r4/Register  init=0  rst=off  en=on  dbl_ovrd=off  block_type=register
      settings: block_version=VER_STRING_GOES_HERE
  Register1 : xbsIndex_r4/Register  init=0  rst=off  en=off  dbl_ovrd=off  block_type=register
      settings: block_version=VER_STRING_GOES_HERE
  Dout : Outport
  Valid : Outport  Port=2
  wires:
  en/1 -> Register1/1, Register/2
  Register1/1 -> Valid/1
  Register/1 -> Dout/1
  Din/1 -> Register/1

== system ddc_bpm_476_066_bak6/Channel3_tbt/decim35/Cast1/format1 ==
  din : Inport
  Convert : xbsIndex_r4/Convert  gui_display_data_type=Fixed-point  arith_type="Signed  (2's comp)"  n_bits=24  bin_pt=22  float_type=Single  exp_bits=8  fraction_bits=24  quantization="Round  (unbiased: +/- Inf)"  overflow=Flag as error  en=off  latency=0  dbl_ovrd=off  pipeline=off  block_type=convert
  Reinterpret : xbsIndex_r4/Reinterpret  force_arith_type=on  arith_type="Signed  (2's comp)"  force_bin_pt=off  bin_pt=22  block_type=reinterpret
      settings: block_version=10.1
  dout : Outport
  wires:
  din/1 -> Reinterpret/1
  Convert/1 -> dout/1
  Reinterpret/1 -> Convert/1

== system ddc_bpm_476_066_bak6/Channel3_tbt/decim35/Cast4/format1 ==
  din : Inport
  Convert : xbsIndex_r4/Convert  gui_display_data_type=Fixed-point  arith_type="Signed  (2's comp)"  n_bits=24  bin_pt=22  float_type=Single  exp_bits=8  fraction_bits=24  quantization="Round  (unbiased: +/- Inf)"  overflow=Flag as error  en=off  latency=0  dbl_ovrd=off  pipeline=off  block_type=convert
  Reinterpret : xbsIndex_r4/Reinterpret  force_arith_type=on  arith_type="Signed  (2's comp)"  force_bin_pt=off  bin_pt=22  block_type=reinterpret
      settings: block_version=10.1
  dout : Outport
  wires:
  din/1 -> Reinterpret/1
  Convert/1 -> dout/1
  Reinterpret/1 -> Convert/1
